simulink model "s_deng_rev1_13_sband"  (R2016b)
(part 4 of 69)

  flag_setup/5(in_reset_flags) -> pipeline36/1(d)
  pipeline36/1(q) -> edge_detect8/1(in)
  pipeline35/1(q) -> edge_detect9/1(in)
  pipeline34/1(q) -> [ndiode_flag]
  pipeline33/1(q) -> [adc_flag]
  pipeline32/1(q) -> [adc_count]
  start_flag_msw/1(in_reg) -> pipeline37/1(d)
  pipeline37/1(q) -> Concat4/1
  start_flag_lsw/1(in_reg) -> pipeline38/1(d)
  pipeline38/1(q) -> Concat4/2
  end_flag_msw/1(in_reg) -> pipeline39/1(d)
  pipeline39/1(q) -> Concat5/1
  end_flag_lsw/1(in_reg) -> pipeline40/1(d)
  pipeline40/1(q) -> Concat5/2
  pipeline54/1(q) -> [spead_data0]  "sp0_data"
  pipeline55/1(q) -> [spead_valid0]  "sp0_valid"
  pipeline56/1(q) -> [spead_eof0]  "sp0_eof"
  pipeline57/1(q) -> [spead_data1]  "sp1_data"
  pipeline58/1(q) -> [spead_valid1]  "sp1_valid"
  pipeline59/1(q) -> [spead_eof1]  "sp1_eof"
  pipeline60/1(q) -> [spead_data2]  "sp2_data"
  pipeline61/1(q) -> [spead_valid2]  "sp2_valid"
  pipeline62/1(q) -> [spead_eof2]  "sp2_eof"
  pipeline63/1(q) -> [spead_data3]  "sp3_data"
  pipeline64/1(q) -> [spead_valid3]  "sp3_valid"
  pipeline65/1(q) -> [spead_eof3]  "sp3_eof"
  pipeline97/1(q) -> Gateway Out70/1, pack_80_64_00/2(valid80)
  pipeline98/1(q) -> Gateway Out71/1, pack_80_64_00/3(word_start)
  pipeline99/1(q) -> Logical18/2, Gateway Out72/1, pack_80_64_00/4(pkt_start)
  pipeline101/1(q) -> Gateway Out73/1, pack_80_64_1/2(valid80)
  pipeline102/1(q) -> Gateway Out74/1, pack_80_64_1/3(word_start)
  pipeline105/1(q) -> Gateway Out76/1, pack_80_64_2/2(valid80)
  pipeline106/1(q) -> Gateway Out77/1, pack_80_64_2/3(word_start)
  pipeline109/1(q) -> Gateway Out79/1, pack_80_64_3/2(valid80)
  pipeline110/1(q) -> Gateway Out80/1, pack_80_64_3/3(word_start)
  pipeline112/1(q) -> Logical42/2, [rdy0], Gateway Out26/1
  pipeline113/1(q) -> Logical43/1, Gateway Out69/1, [vld0], Gateway Out25/1
  pipeline115/1(q) -> Logical11/2, [rdy1]
  pipeline116/1(q) -> Logical41/2, [vld1]
  pipeline118/1(q) -> Logical44/2, [rdy2]
  pipeline119/1(q) -> Logical45/1, [vld2]
  pipeline121/1(q) -> Logical46/2, [rdy3]
  pipeline122/1(q) -> Logical47/1, [vld3]
  Delay13/1 -> Logical8/1, Logical6/1
  Delay14/1 -> Logical7/2
  Delay15/1 -> Delay18/1
  Delay16/1 -> Delay19/1
  Delay17/1 -> Logical5/1
  Delay18/1 -> Delay20/1
  Delay19/1 -> Delay21/1
  Delay20/1 -> sample_masking/3(first_samples)
  Delay21/1 -> sample_masking/4(last_samples)
  Delay22/1 -> Logical3/2
  Delay23/1 -> Logical1/1
  Delay24/1 -> Delay25/1
  Delay25/1 -> Delay26/1
  Delay26/1 -> Delay27/1
  Delay27/1 -> sample_masking/1(timei)
  sample_masking/4(flag_valid) -> Delay28/1
  Delay28/1 -> [flag_en]
  Logical1/1 -> sample_masking/7(flag_en)  "flag_en"
  sample_masking/1(timeo) -> Delay29/1
  Delay29/1 -> [masked_time]
  [local_time] -> Delay30/1
  [en_armed] -> Delay31/1
  [local_time] -> Delay32/1, Delay34/1, Delay38/1, Delay40/1
  [start_time] -> Delay33/1
  [end_time] -> Delay35/1, Delay36/1
  Delay30/1 -> Delay24/1
  Delay31/1 -> Delay13/1
  Delay32/1 -> Relational3/1
  Delay33/1 -> Relational3/2
  Delay34/1 -> Relational4/1
  Delay35/1 -> Relational4/2
  Delay36/1 -> Relational5/1
  Delay37/1 -> Relational5/2
  Delay38/1 -> Relational6/1
  Delay39/1 -> Relational6/2
  Delay40/1 -> Relational7/1
  Delay41/1 -> Relational7/2
  Delay44/1 -> Logical4/1, Logical2/1
  Delay45/1 -> Relational/1
  Delay46/1 -> Relational/2
  Delay47/1 -> Relational1/1
  Delay48/1 -> Relational1/2
  Delay51/1 -> Relational2/1
  pipeline127/1(q) -> [pol0_always_on]
  [pol0_always_on] -> gbe0_traffic_control/1(always_on)
  [pol0_requested_pkts] -> gbe0_traffic_control/2(requested_pkts)
  [pol0_offset_data] -> gbe0_traffic_control/3(offset_data)
  [mrst] -> gbe0_traffic_control/4(mrst)
  [pol0_traffic_trigger] -> gbe0_traffic_control/5(traffic_trigger)
  gbe0_traffic_control/1(gbe_txen_gate) -> [gbe_txen_gate0]
  Constant68/1 -> pol1_sample_offset/1(sim_1)
  pipeline129/1(q) -> [pol1_offset_data]
  Constant67/1 -> pol0_sample_offset/1(sim_1)
  pipeline128/1(q) -> [pol0_offset_data]
  Constant69/1 -> pol0_num_pkts/1(sim_1)
  pipeline126/1(q) -> [pol0_requested_pkts]
  Constant73/1 -> pol1_num_pkts/1(sim_1)
  pipeline134/1(q) -> [pol1_requested_pkts]
  pipeline136/1(q) -> [pol1_always_on]
  pipeline5/1(q) -> [gbe_txen]
  Delay/1 -> pol_traffic_trigger/1(sim_1)
  Constant66/1 -> pol_tx_always_on/1(sim_1)
  Constant77/1 -> pol_tx_always_on/2(sim_2)
  pol0_num_pkts/1(in_pol0_num_pkts) -> pipeline126/1(d)
  pol1_num_pkts/1(in_pol1_num_pkts) -> pipeline134/1(d)
  pol_tx_always_on/1(in_pol0_tx_always_on) -> pipeline127/1(d)
  pol_tx_always_on/2(in_pol1_tx_always_on) -> pipeline136/1(d)
  pol0_sample_offset/1(in_pol0_sample_offset) -> pipeline128/1(d)
  pol1_sample_offset/1(in_pol1_sample_offset) -> pipeline129/1(d)
  Delay52/1 -> pol_traffic_trigger/2(sim_2)
  pol_traffic_trigger/1(in_pol0_tx_trigger) -> pipeline131/1(d)
  pipeline130/1(q) -> [pol1_traffic_trigger]
  pol_traffic_trigger/2(in_pol1_tx_trigger) -> pipeline130/1(d)
  edge_detect3/1(out) -> [cnt_rst]  "mrst"
  AddSub/1 -> Slice/1
  AddSub1/1 -> Slice1/1
  [tvg_stime] -> AddSub1/1, AddSub/1
  Constant81/1 -> speadtime0_offset/1(sim_1)
  Slice/1 -> Register5/1
  Slice1/1 -> Register6/1
  speadtime0_offset/1(in_speadtime_offset0) -> AddSub/2
  Constant82/1 -> speadtime1_offset/1(sim_1)
  speadtime1_offset/1(in_speadtime_offset1) -> AddSub1/2
  pipeline131/1(q) -> [pol0_traffic_trigger]
  gbe1_traffic_control/1(gbe_txen_gate) -> [gbe_txen_gate1]
  gbe2_traffic_control/1(gbe_txen_gate) -> [gbe_txen_gate2]
  gbe3_traffic_control/1(gbe_txen_gate) -> [gbe_txen_gate3]
  [spead_valid0] -> gbe0_traffic_control/6(spead_valid)
  [pol0_always_on] -> gbe1_traffic_control/1(always_on)
  [pol0_requested_pkts] -> gbe1_traffic_control/2(requested_pkts)
  [pol0_offset_data] -> gbe1_traffic_control/3(offset_data)
  [mrst] -> gbe1_traffic_control/4(mrst)
  [pol0_traffic_trigger] -> gbe1_traffic_control/5(traffic_trigger)
  [pol1_always_on] -> gbe2_traffic_control/1(always_on)
  [pol1_requested_pkts] -> gbe2_traffic_control/2(requested_pkts)
  [pol1_offset_data] -> gbe2_traffic_control/3(offset_data)
  [mrst] -> gbe2_traffic_control/4(mrst)
  [pol1_traffic_trigger] -> gbe2_traffic_control/5(traffic_trigger)
  [pol1_always_on] -> gbe3_traffic_control/1(always_on)
  [pol1_requested_pkts] -> gbe3_traffic_control/2(requested_pkts)
  [pol1_offset_data] -> gbe3_traffic_control/3(offset_data)
  [mrst] -> gbe3_traffic_control/4(mrst)
  [pol1_traffic_trigger] -> gbe3_traffic_control/5(traffic_trigger)
  [spead_valid1] -> gbe1_traffic_control/6(spead_valid)
  [spead_valid2] -> gbe2_traffic_control/6(spead_valid)
  [spead_valid3] -> gbe3_traffic_control/6(spead_valid)
  Constant59/1 -> Delay/1
  Constant40/1 -> Delay52/1
  master_reset_sim7/1 -> dram_addr_offset/1(sim_1)
  master_reset_sim8/1 -> arb_rst/1(sim_1)
  master_reset_sim9/1 -> arb_en/1(sim_1)
  pipeline133/1(q) -> [arb_en0]
  pipeline138/1(q) -> [dram_addr_offset0]
  master_reset_sim1/1 -> dram_read_length/1(sim_1)
  master_reset_sim2/1 -> dram_rd_trigger/1(sim_1)
  pipeline150/1(q) -> [dram_rd_trig0]
  master_reset_sim3/1 -> dram_tvg/1(sim_1)
  master_reset_sim4/1 -> dram_tvg_length/1(sim_1)
  pipeline148/1(q) -> [dram_tvg_length0]
  edge_detect13/1(out) -> [arb_rst0]
  pipeline135/1(q) -> edge_detect13/1(in)
  master_reset_sim5/1 -> dram_rd_repeat/1(sim_1)
  pipeline151/1(q) -> [dram_rd_repeat0]
  pipeline146/1(q) -> Slice13/1, Slice11/1
  Slice13/1 -> Logical17/1, [tvg_sel0]
  Slice11/1 -> Logical17/2
  Logical17/1 -> [dram_tvg0]
  pipeline149/1(q) -> [dram_read_length0]
  master_reset_sim6/1 -> dram_rd_repeat_rate/1(sim_1)
  pipeline137/1(q) -> [dram_rd_repeat_delay0]
  [cwg_80_0] -> pipeline190/1(d)
  pipeline158/1(q) -> [source_sel_0]
  pipeline159/1(q) -> [source_sel_1]
  Constant87/1 -> src_sel_cntrl/1(sim_1)
  Constant88/1 -> src_sel_cntrl/2(sim_2)
  src_sel_cntrl/1(in_src_sel_0) -> pipeline158/1(d)
  src_sel_cntrl/2(in_src_sel_1) -> pipeline159/1(d)
  [source_sel_0] -> pipeline189/1(d)
  Inverter/1 -> fifo1/2(fifo_we_en)
  Gateway Out24/1 -> To Workspace24/1
  Slice23/1 -> Gateway Out24/1
  Gateway Out25/1 -> To Workspace25/1
  Gateway Out26/1 -> To Workspace26/1
  dram_rd_repeat_rate/1(in_dram_rd_repeat_rate) -> pipeline137/1(d)
  dram_rd_repeat/1(in_dram_rd_repeat) -> pipeline151/1(d)
  dram_tvg/1(in_arb_tvg) -> pipeline146/1(d)
  dram_tvg_length/1(in_tvg_length) -> pipeline148/1(d)
  dram_addr_offset/1(in_dram_addr_offset) -> pipeline138/1(d)
  dram_read_length/1(in_dram_read_length) -> pipeline149/1(d)
  dram_rd_trigger/1(in_arb_trig) -> pipeline150/1(d)
  arb_en/1(in_arb_en) -> pipeline133/1(d)
  arb_rst/1(in_rst) -> pipeline135/1(d)
  pipeline189/1(q) -> Mux5/1
  pipeline190/1(q) -> Mux5/2
  pipeline191/1(q) -> Mux5/3
  [adc_count] -> Concat6/1
  Constant90/1 -> Concat6/2
  Delay4/1 -> [status0]
  Delay55/1 -> [status3]
  Delay54/1 -> [status2]
  Delay53/1 -> [status1]
  Concat6/1 -> Delay55/1, Delay4/1, Delay53/1, Delay54/1
  [ndiode_flag] -> Convert28/1
  Logical/1 -> Convert27/1
  Logical19/1 -> Convert30/1
  [adc_flag] -> Convert29/1
  [flag_en] -> Logical/1, Logical19/2
  Convert28/1 -> Logical/2
  Convert29/1 -> Logical19/1
  Convert30/1 -> Concat6/3
  Convert27/1 -> Concat6/4
  Gateway Out13/1 -> To Workspace13/1
  [local_time] -> pipeline203/1(d)
  [mrst] -> pipeline201/1(d)
  [wng_man_rst0] -> pipeline199/1(d)
  wng_rst/1(wng_rst) -> Gateway Out13/1, [wng_rst0]
  Constant89/1 -> rpt_length_wng0/1(sim_1)
  pipeline200/1(q) -> wng_rst/5(num_samples_for_rst)
  pipeline199/1(q) -> wng_rst/4(man_rst)
  pipeline201/1(q) -> wng_rst/3(mrst)
  pipeline202/1(q) -> wng_rst/2(future_time)
  pipeline203/1(q) -> wng_rst/1(local_time)
  Constant95/1 -> rpt_load_time_msw_wng0/1(sim_1)
  Constant93/1 -> rpt_load_time_lsw_wng0/1(sim_1)
  Concat3/1 -> Delay1/1
  pipeline204/1(q) -> Concat3/1
  pipeline205/1(q) -> Concat3/2
  rpt_load_time_lsw_wng0/1(in_reg) -> pipeline205/1(d)
  rpt_load_time_msw_wng0/1(in_reg) -> pipeline204/1(d)
  Delay1/1 -> pipeline202/1(d)
  rpt_length_wng0/1(in_samples) -> pipeline206/1(d)
  pipeline206/1(q) -> pipeline200/1(d)
  [local_time] -> pipeline154/1(d)
  impulse/1(impulse0) -> [impulse_gen0]
  pipeline152/1(q) -> impulse/2(future_time)
  pipeline154/1(q) -> impulse/1(local_time)
  Constant92/1 -> impulse_load_time_msw/1(sim_1)
  Constant91/1 -> impulse_load_time_lsw/1(sim_1)
  Concat7/1 -> Delay10/1
  pipeline155/1(q) -> Concat7/1
  pipeline160/1(q) -> Concat7/2
  impulse_load_time_lsw/1(in_reg) -> pipeline160/1(d)
  impulse_load_time_msw/1(in_reg) -> pipeline155/1(d)
  Delay10/1 -> pipeline152/1(d)
  pipeline163/1(q) -> Mux5/4
  [impulse_gen0] -> pipeline163/1(d)
  gpio/1 -> Terminator62/1
  Gateway Out/1 -> To Workspace/1
  impulse/2(impulse_gpio) -> [impulse_gpio]
  pipeline145/1(q) -> impulse/3(delay_correction)
  impulse_delay_correction/1(in_reg) -> pipeline145/1(d)
  Constant55/1 -> impulse_delay_correction/1(sim_1)
  pipeline144/1(q) -> Gateway Out/1, gpio/1
  [impulse_gpio] -> pipeline144/1(d)
  bus_create4/1(bus_out) -> pipeline191/1(d)
  [tvg_ltime] -> Delay11/1
  Delay11/1 -> Delay12/1
  [data_80_0] -> Delay56/1
  Delay56/1 -> Delay57/1
  bus_expand14/7(out2) -> pipeline167/1(d)
  bus_expand14/8(lsb_out1) -> pipeline170/1(d)
  bus_expand14/6(out3) -> pipeline171/1(d)
  bus_expand14/5(out4) -> pipeline172/1(d)
  bus_expand14/4(out5) -> pipeline209/1(d)
  bus_expand14/3(out6) -> pipeline210/1(d)
  bus_expand14/2(out7) -> pipeline211/1(d)
  bus_expand14/1(msb_out8) -> pipeline212/1(d)
  pipeline212/1(q) -> ss_fifo_in/1(in_d0)
  pipeline211/1(q) -> ss_fifo_in/2(in_d1)
  pipeline210/1(q) -> ss_fifo_in/3(in_d2)
  pipeline209/1(q) -> ss_fifo_in/4(in_d3)
  pipeline172/1(q) -> ss_fifo_in/5(in_d4)
  pipeline171/1(q) -> ss_fifo_in/6(in_d5)
  pipeline167/1(q) -> ss_fifo_in/7(in_d6)
  pipeline170/1(q) -> ss_fifo_in/8(in_d7)
  Delay57/1 -> bus_expand14/1(bus_in)
  Delay12/1 -> pipeline215/1(d), Relational8/1
  pipeline215/1(q) -> ss_localtime/1(in_time)
  pipeline213/1(q) -> ss_fifo_in/9(in_gpio_trig)
  Delay58/1 -> Delay59/1
  Delay59/1 -> pipeline213/1(d)
  [impulse_gpio] -> Delay60/1
  Delay60/1 -> Delay58/1
  pipeline214/1(q) -> impulse/4(Impulse_offset)
  Constant109/1 -> impulse_offset/1(sim_1)
  impulse_offset/1(in_reg) -> pipeline214/1(d)
  Constant108/1 -> ss_trig_time_msw/1(sim_1)
  Constant107/1 -> ss_trig_time_lsw/1(sim_1)
  Concat8/1 -> Delay61/1
  pipeline216/1(q) -> Concat8/1
  pipeline217/1(q) -> Concat8/2
  ss_trig_time_lsw/1(in_reg) -> pipeline217/1(d)
  ss_trig_time_msw/1(in_reg) -> pipeline216/1(d)
  Delay61/1 -> Relational8/2
  Relational8/1 -> edge_detect/1
  pipeline218/1(q) -> ss_fifo_in/10(we)
  [fifoselect] -> pipeline219/1(d), pipeline218/1(d)
  pipeline219/1(q) -> ss_localtime/2(we)
  edge_detect/1 -> ss_localtime/3(trig), ss_fifo_in/11(trig)
  Constant111/1 -> start_load_time_msw/1(sim_1)
  Constant110/1 -> start_load_time_lsw/1(sim_1)
  pipeline220/1(q) -> Concat9/1
  pipeline221/1(q) -> Concat9/2
  start_load_time_msw/1(in_reg) -> pipeline220/1(d)
  start_load_time_lsw/1(in_reg) -> pipeline221/1(d)
  Concat9/1 -> Delay62/1
  Constant113/1 -> stop_load_time_msw/1(sim_1)
  Constant112/1 -> stop_load_time_lsw/1(sim_1)
  pipeline222/1(q) -> Concat10/1
  pipeline223/1(q) -> Concat10/2
  stop_load_time_msw/1(in_reg) -> pipeline222/1(d)
  stop_load_time_lsw/1(in_reg) -> pipeline223/1(d)
  Concat10/1 -> Delay63/1
  Delay62/1 -> pipeline225/1(d)
  Delay63/1 -> pipeline224/1(d)
  pipeline225/1(q) -> start_stop_cntrl/1(start_time)
  pipeline224/1(q) -> start_stop_cntrl/2(stop_time)
  [mrst] -> start_stop_cntrl/3(rst)
  start_stop_cntrl/1(start_stop_sel) -> [start_stop_sel]
  pipeline195/1(q) -> Mux3/2
  Mux3/1 -> [data_80_0]
  [start_stop_sel] -> Mux3/1
  Constant115/1 -> Mux3/3
  data_ins/1(data) -> Delay73/1
  debug_control/1(in_reg) -> Slice2/1, Slice10/1
  Constant94/1 -> debug_control/1(sim_1)
  Constant120/1 -> pkt_size0/1(sim_1)
  pkt_size0/1(in_reg) -> Delay67/1, Relational9/1
  pkt_size_calc0/1(en_out) -> Delay69/1
  pkt_size_calc0/2(eof) -> Delay70/1
  data_ins/2(en_out) -> Delay74/1
  data_ins/3(eof_out) -> Delay75/1
  [debug_cnt_rst] -> data_ins/1(rst)
  Slice2/1 -> Delay64/1
  Delay64/1 -> [debug_cnt_rst]
  Gateway Out8/1 -> Scope1/1
  Gateway Out10/1 -> Scope1/2
  Gateway Out11/1 -> Scope1/3
  Gateway Out14/1 -> Scope1/4
  Slice3/1 -> Gateway Out8/1
  Slice4/1 -> Gateway Out10/1
  Logical22/1 -> Counter1/2, Gateway Out7/1
  Counter1/1 -> Delay68/1, Gateway Out2/1
  [debug_cnt_rst] -> Counter1/1
  Delay67/1 -> pkt_size_calc0/2(size)
  Delay68/1 -> Convert10/1
  Delay69/1 -> data_ins/2(en_in)
  Delay70/1 -> data_ins/3(eof_in)
  Delay71/1 -> pkt_size_calc0/3(en_in)
  Delay73/1 -> Slice3/1, Slice4/1
  Delay74/1 -> Gateway Out11/1, Logical22/1
  Delay75/1 -> Gateway Out14/1, Logical22/2
  Slice10/1 -> Delay81/1
  pkt_rate0/1(en) -> Delay83/1, Logical23/3
  Logical23/1 -> Delay71/1
  Delay81/1 -> Logical23/2
  Gateway Out2/1 -> Scope4/1
  Gateway Out7/1 -> Scope4/2
  Counter3/1 -> Delay82/1
  Delay82/1 -> debug_rate/1(out_reg)
  Delay83/1 -> Counter3/1
  Constant119/1 -> Relational9/2
  Relational9/1 -> Logical23/1
  [debug_cnt_rst] -> pkt_size_calc0/1(rst)
  Convert10/1 -> debug_tx_pkt_cnt/1(out_reg)
  [forty_gbe_led_up] -> Delay72/1
  [forty_gbe_led_rx] -> Delay101/1
  [forty_gbe_led_tx] -> Delay110/1
  [forty_gbe_tx_afull] -> Delay107/1
  [forty_gbe_tx_overflow] -> Delay112/1
  [forty_gbe_rx_overrun] -> Delay111/1
  [arb_rst0] -> Terminator9/1
  [arb_en0] -> Terminator10/1
  [dram_rd_repeat0] -> Terminator11/1
  [dram_rd_repeat_delay0] -> Terminator13/1
  [tvg_sel0] -> Terminator14/1
  [dram_tvg0] -> Terminator17/1
  [dram_tvg_length0] -> Terminator19/1
  [dram_addr_offset0] -> Terminator21/1
  [dram_read_length0] -> Terminator22/1
  Delay107/1 -> status0/4(out_tx_afull)
  Delay101/1 -> status0/2(out_led_rx)
  Delay112/1 -> status0/5(out_tx_overflow)
  Delay111/1 -> status0/6(out_rx_overrun)
  Delay110/1 -> status0/3(out_led_tx)
  Delay72/1 -> status0/1(out_led_up)
  pipeline15/1(q) -> [gbe_port]
  Constant26/1 -> [spead_heapsize]
  Constant27/1 -> [spead_pktlen]
  Constant45/1 -> [spead_heapoffset]
  Constant8/1 -> [adc_data_offset]
  [spead_data0] -> pipeline72/1(d)
  [spead_valid0] -> pipeline73/1(d)
  wr_addr0/1 -> Gateway Out63/1, 64_to_256/1  "waddr"
  [spead_valid0] -> Gateway Out19/1, edge_detect27/1(in), edge_detect7/1, pipeline67/1(d)
  Constant116/1 -> 64_to_256/6
  Constant121/1 -> 64_to_256/5
  rd_addr0/1 -> Gateway Out64/1, 64_to_256/4, Relational13/2  "rdaddr"
  edge_detect7/1 -> wr_addr0/1
  pipeline67/1(q) -> wr_addr0/2
  pipeline72/1(q) -> 64_to_256/2
  pipeline73/1(q) -> 64_to_256/3  "dv64_0"
  64_to_256/1 -> Terminator25/1
  edge_detect27/1(out) -> rd_addr0/1, rd_arm/3, rd_arm/1
  Constant131/1 -> Relational13/1
  Relational13/1 -> rd_arm/2  "rd_done"
  rd_arm/1 -> pipeline74/1(d), rd_addr0/2  "rd_en"
  edge_detect17/1(out) -> [sp256_eof0]  "eof256_0"
  [spead_data2] -> pipeline77/1(d)
  [spead_valid2] -> pipeline80/1(d)
  wr_addr2/1 -> 64_to_1/1  "waddr"
  [spead_valid2] -> pipeline76/1(d), edge_detect18/1, edge_detect20/1(in), Gateway Out21/1
  Constant21/1 -> 64_to_1/6
  Constant25/1 -> 64_to_1/5
  rd_addr2/1 -> Relational14/2, 64_to_1/4  "rdaddr"
  edge_detect18/1 -> wr_addr2/1
  pipeline76/1(q) -> wr_addr2/2
  pipeline77/1(q) -> 64_to_1/2
  pipeline80/1(q) -> 64_to_1/3  "dv64_2"
  64_to_1/1 -> Terminator26/1
  edge_detect20/1(out) -> rd_addr2/1
  Constant86/1 -> Relational14/1
  Relational14/1 -> rd_arm2/2  "rd_done"
  rd_arm2/1 -> rd_addr2/2, pipeline81/1(d)  "rd_en"
  pipeline81/1(q) -> edge_detect19/1(in), pipeline82/1(d)  "dv256"
  edge_detect19/1(out) -> [sp256_eof2]  "eof256_2"
  pipeline82/1(q) -> [sp256_dv2]  "dv256_2"
  [sp256_eof0] -> rd_arm2/3, rd_arm2/1
  [spead_data1] -> pipeline84/1(d)
  [spead_valid1] -> pipeline85/1(d)
  wr_addr1/1 -> 64_to_2/1  "waddr"
  [spead_valid1] -> pipeline83/1(d), edge_detect21/1, Gateway Out20/1, edge_detect23/1(in)
  Constant122/1 -> 64_to_2/6
  Constant123/1 -> 64_to_2/5
  rd_addr1/1 -> Relational10/2, 64_to_2/4  "rdaddr"
  edge_detect21/1 -> wr_addr1/1
  pipeline83/1(q) -> wr_addr1/2
  pipeline84/1(q) -> 64_to_2/2
  pipeline85/1(q) -> 64_to_2/3  "dv64_1"
  64_to_2/1 -> Terminator27/1
  edge_detect23/1(out) -> rd_arm1/3, rd_arm1/1, rd_addr1/1
  Constant124/1 -> Relational10/1
  Relational10/1 -> rd_arm1/2  "rd_done"
  rd_arm1/1 -> rd_addr1/2, pipeline86/1(d)  "rd_en"
  pipeline86/1(q) -> edge_detect22/1(in), pipeline124/1(d)  "dv256"
  edge_detect22/1(out) -> [sp256_eof1]  "eof256_1"
  pipeline124/1(q) -> [sp256_dv1]  "dv256_1"
  [spead_data3] -> pipeline132/1(d)
  [spead_valid3] -> pipeline139/1(d)
  wr_addr3/1 -> 64_to_3/1  "waddr"
  [spead_valid3] -> edge_detect26/1(in), Gateway Out22/1, edge_detect24/1, pipeline125/1(d)
  Constant125/1 -> 64_to_3/6
  Constant126/1 -> 64_to_3/5
  rd_addr3/1 -> 64_to_3/4, Relational11/2  "rdaddr"
  edge_detect24/1 -> wr_addr3/1
  pipeline125/1(q) -> wr_addr3/2
  pipeline132/1(q) -> 64_to_3/2
  pipeline139/1(q) -> 64_to_3/3  "dv64_3"
  64_to_3/1 -> Terminator24/1
  edge_detect26/1(out) -> rd_addr3/1
  Constant127/1 -> Relational11/1
  Relational11/1 -> rd_arm3/2  "rd_done"
  rd_arm3/1 -> pipeline140/1(d), rd_addr3/2  "rd_en"
  pipeline140/1(q) -> edge_detect25/1(in), pipeline141/1(d)  "dv256"
  edge_detect25/1(out) -> [sp256_eof3]  "eof256_3"
  pipeline141/1(q) -> [sp256_dv3]  "dv256_3"
  [sp256_eof1] -> rd_arm3/1, rd_arm3/3
  [gbe_txen0] -> Logical12/2
  pipeline75/1(q) -> [sp256_dv0]  "dv256_0"
  [sp256_eof0] -> Logical12/1
  [sp256_dv0] -> Logical13/1
  [gbe_txen0] -> Logical13/2
  Logical13/1 -> Gateway Out65/1, [sp256_dvg0]
  Logical12/1 -> Gateway Out90/1, [sp256_eofg0]
  [gbe_txen1] -> Logical14/2
  [sp256_eof1] -> Logical14/1
  [sp256_dv1] -> Logical15/1
  [gbe_txen1] -> Logical15/2
  Logical15/1 -> Gateway Out66/1, [sp256_dvg1]
  Logical14/1 -> Gateway Out89/1, [sp256_eofg1]
  [gbe_txen2] -> Logical16/2
  [sp256_eof2] -> Logical16/1
  [sp256_dv2] -> Logical25/1
  [gbe_txen2] -> Logical25/2
  Logical25/1 -> Gateway Out67/1, [sp256_dvg2]
  Logical16/1 -> Gateway Out88/1, [sp256_eofg2]
  [gbe_txen3] -> Logical26/2
  [sp256_eof3] -> Logical26/1
  [sp256_dv3] -> Logical27/1
  [gbe_txen3] -> Logical27/2
  Logical27/1 -> Gateway Out68/1, [sp256_dvg3]
  Logical26/1 -> Gateway Out87/1, [sp256_eofg3]
  [sel_munge] -> Mux17/1
  Mux17/1 -> [sp256_data3]
  [sel_munge] -> Mux16/1
  Mux16/1 -> [sp256_data2]
  [sel_munge] -> Mux18/1
  Mux18/1 -> [sp256_data1]
  [sel_munge] -> Mux19/1
  Mux19/1 -> [sp256_data0]
  [gbe_rst] -> pipeline233/1(d)
  Constant18/1 -> forty_gbe/7(rx_ack)
  Constant56/1 -> forty_gbe/8(rx_overrun_ack)
  pipeline239/1(q) -> forty_gbe/9(debug_rst)
  Logical40/1 -> pipeline238/1(d)
  Logical39/1 -> pipeline235/1(d)
  [sp256_data] -> pipeline234/1(d)
  [gbe_port] -> pipeline237/1(d)
  [gbe_txip] -> pipeline236/1(d)
  forty_gbe/1(led_up) -> pipeline178/1(d)
  forty_gbe/2(led_rx) -> pipeline87/1(d)
  forty_gbe/3(led_tx) -> pipeline176/1(d)
  forty_gbe/4(tx_afull) -> pipeline177/1(d)
  forty_gbe/5(tx_overflow) -> pipeline179/1(d)
  forty_gbe/12(rx_overrun) -> pipeline197/1(d)
  forty_gbe/6(rx_data) -> Terminator42/1
  forty_gbe/7(rx_valid) -> Terminator43/1
  forty_gbe/10(rx_end_of_frame) -> Terminator44/1
  forty_gbe/11(rx_bad_frame) -> Terminator45/1
  forty_gbe/8(rx_source_ip) -> Terminator7/1
  forty_gbe/9(rx_source_port) -> Terminator8/1
  pipeline178/1(q) -> [forty_gbe_led_up]
  pipeline87/1(q) -> [forty_gbe_led_rx]
  pipeline176/1(q) -> [forty_gbe_led_tx]
  pipeline177/1(q) -> [forty_gbe_tx_afull]
  pipeline179/1(q) -> [forty_gbe_tx_overflow]
  pipeline197/1(q) -> [forty_gbe_rx_overrun]
  forty_gbe/14(rx_dest_port) -> Terminator40/1
  forty_gbe/13(rx_dest_ip) -> Terminator41/1
  [gbe_txen] -> Logical39/1
  [sp256_dv] -> Logical39/2
  [gbe_txen] -> Logical40/1
  [sp256_eof] -> Logical40/2
  pipeline233/1(q) -> forty_gbe/1(rst)
  pipeline234/1(q) -> forty_gbe/2(tx_data)
  pipeline235/1(q) -> forty_gbe/3(tx_valid)
  pipeline236/1(q) -> forty_gbe/4(tx_dest_ip)
  pipeline237/1(q) -> forty_gbe/5(tx_dest_port)
  pipeline238/1(q) -> forty_gbe/6(tx_end_of_frame)
  [cnt_rst] -> pipeline239/1(d)
  ramp0/1 -> [rampdata0]
  [vld0] -> ramp0/2
  [rdy0] -> ramp0/1
  ramp1/1 -> [rampdata1]
  [vld1] -> ramp1/2
  [rdy1] -> ramp1/1
  [spead_data0] -> spead_snap0/1(in_d64)
  [spead_valid0] -> spead_snap0/2(we)
  [spead_eof0] -> spead_detail/1(in_eof)
  [spead_valid0] -> spead_detail/2(in_we), spead_detail/3(we)
  Logical9/1 -> spead_detail/4(trig), spead_snap0/3(trig)
  [spead_eof0] -> Logical9/2
  [speadsnap_arm] -> Logical9/1
  speadsnap_control/1(in_speadsnap_arm) -> Delay65/1
  Delay65/1 -> [speadsnap_arm]
  ramp2/1 -> [rampdata2]
  [vld2] -> ramp2/2
  [rdy2] -> ramp2/1
  ramp3/1 -> [rampdata3]
  [vld3] -> ramp3/2
  [rdy3] -> ramp3/1
  ramp80/1 -> [ramp79]
  [rst_ramp80] -> ramp80/1
  Delay76/1 -> [sel_ramp80]
  ramp_control/1(in_sel_ramp80) -> Delay76/1
  Delay77/1 -> [rst_ramp80]
  ramp_control/2(in_rst_ramp80) -> Delay77/1
  Delay66/1 -> [sel_munge]
  ramp_control/3(in_sel_munge) -> Delay66/1
  gbe_control/1(in_gbe0) -> [gbe_txen0]
  gbe_control/2(in_gbe1) -> [gbe_txen1]
  gbe_control/3(in_gbe2) -> [gbe_txen2]
  gbe_control/4(in_gbe3) -> [gbe_txen3]
  Constant117/1 -> gbe_control/2(sim_2)
  Constant65/1 -> gbe_control/1(sim_1)
  Constant118/1 -> gbe_control/3(sim_3)
  Constant132/1 -> gbe_control/4(sim_4)
  pipeline68/1(q) -> Mux14/2
  [sel_ramp80] -> Mux14/1
  Mux14/1 -> Slice23/1, Gateway Out107/1, spead_pack0/3(data64)
  pack_80_64_00/3(data64) -> pipeline68/1(d)  "d64_00"
  [sel_ramp80] -> Mux15/1
  Mux15/1 -> Gateway Out108/1, spead_pack1/3(data64)
  [sel_ramp80] -> Mux20/1
  Mux20/1 -> Gateway Out109/1, spead_pack2/3(data64)
  [sel_ramp80] -> Gateway Out113/1, Mux21/1
  [ramp79] -> bus_create4/2(in2)  "d80_0"
  Constant133/1 -> bus_create4/1(in1)
  [rampdata0] -> Mux14/3
  [rampdata1] -> Mux15/3
  pipeline117/1(q) -> Mux15/2
  [rampdata2] -> Mux20/3
  pipeline120/1(q) -> Mux20/2
  [rampdata3] -> Mux21/3
  pipeline123/1(q) -> Mux21/2
  Logical11/1 -> spead_pack1/1(data64_ready)
  Logical41/1 -> spead_pack1/2(data64_valid), Gateway Out62/1
  [gbe_txen_gate1] -> Logical41/1, Logical11/1
  [gbe_txen_gate0] -> Logical43/2, Gateway Out60/1, Logical42/1
  Logical43/1 -> Gateway Out61/1, spead_pack0/2(data64_valid)
  Logical42/1 -> spead_pack0/1(data64_ready)
  [gbe_txen_gate2] -> Logical45/2, Logical44/1
  Logical44/1 -> spead_pack2/1(data64_ready)
  Logical45/1 -> spead_pack2/2(data64_valid), Gateway Out85/1
  [gbe_txen_gate3] -> Logical47/2, Logical46/1
  Logical46/1 -> spead_pack3/1(data64_ready)
  Logical47/1 -> spead_pack3/2(data64_valid), Gateway Out86/1
  bram_munge0/1(Out1) -> Mux19/2
  bram_munge1/1(Out1) -> Mux18/2
  bram_munge2/1(Out1) -> Mux16/2
  bram_munge3/1(Out1) -> Mux17/2
  Delay78/1 -> Mux9/1
  [speadtime0] -> Mux9/3
  pipeline96/1(q) -> Mux9/2
  Mux9/1 -> pack_80_64_00/1(data80)
  Logical18/1 -> Delay78/1
  [sel_insert_time] -> Logical18/1
  [mrst] -> Gateway Out98/1, ticks_since_mrst/1(reset)
  [msync] -> Gateway Out99/1, ticks_since_mrst/2(sync)
  control/1(in_cnt_rst) -> pipeline/1(d)
  ramp_control/4(in_sel_insert_time) -> Delay79/1
  Delay79/1 -> [sel_insert_time]
  pipeline103/1(q) -> Logical48/2, Gateway Out75/1, pack_80_64_1/4(pkt_start)
  Delay80/1 -> Mux10/1
  Logical48/1 -> Delay80/1
  [sel_insert_time] -> Logical48/1
  [speadtime1] -> Mux10/3
  pipeline100/1(q) -> Mux10/2
  Mux10/1 -> pack_80_64_1/1(data80)
  Delay84/1 -> Mux22/1
  Logical49/1 -> Delay84/1
  [sel_insert_time] -> Logical49/1
  Mux22/1 -> pack_80_64_2/1(data80)
  [speadtime0] -> Mux22/3
  pipeline104/1(q) -> Mux22/2
  pipeline111/1(q) -> Logical50/2, Gateway Out81/1, pack_80_64_3/4(pkt_start)
  Delay85/1 -> Mux23/1
  Logical50/1 -> Delay85/1
  [sel_insert_time] -> Logical50/1
  Mux23/1 -> pack_80_64_3/1(data80)
  [speadtime1] -> Mux23/3
  pipeline108/1(q) -> Mux23/2
  [start_stop_sel] -> Counter4/2
  Counter4/1 -> start_stop_ctr/1(out_reg)
  [cnt_rst] -> Counter4/1
  [gbe_txen_gate0] -> Counter5/2
  Counter5/1 -> tx_gate_ctrs/1(out_sp0)
  [cnt_rst] -> Counter6/1, Counter7/1, Counter8/1, Counter5/1
  Counter6/1 -> tx_gate_ctrs/2(out_sp1)
  Counter7/1 -> tx_gate_ctrs/3(out_sp2)
  Counter8/1 -> tx_gate_ctrs/4(out_sp3)
  [gbe_txen_gate3] -> Counter8/2
  [gbe_txen_gate2] -> Counter7/2
  [gbe_txen_gate1] -> Counter6/2
  Mux5/1 -> pipeline195/1(d)
  [cwg_80_1] -> pipeline114/1(d)
  [source_sel_1] -> pipeline71/1(d)
  pipeline71/1(q) -> Mux25/1
  pipeline114/1(q) -> Mux25/2
  pipeline142/1(q) -> Mux25/3
  pipeline70/1(q) -> Mux25/4
  [impulse_gen0] -> pipeline70/1(d)
  bus_create5/1(bus_out) -> pipeline142/1(d)
  pipeline143/1(q) -> Mux6/2
  [start_stop_sel] -> Mux6/1
  Constant20/1 -> Mux6/3
  [ramp79] -> bus_create5/2(in2)  "d80_0"
  Constant24/1 -> bus_create5/1(in1)
  Mux25/1 -> pipeline143/1(d)
  scale_wng1/1(in_scale) -> Gateway Out6/1, pipeline47/1(d)
  scale_wng_corr/1(in_scale) -> pipeline46/1(d)
  [wng0_tp0] -> pipeline91/1(d)
  [wng1_tp0] -> pipeline94/1(d)
  cwg_corr/1(bus_out) -> pipeline90/1(d)
  bus_addsub2/1(dout) -> Delay8/1
  bus_addsub4/1(dout) -> bus_convert6/1(din)
  bus_mult/1(a*b) -> [cwg0_tp1], bus_convert/1(din)
  bus_addsub5/1(dout) -> bus_convert7/1(din)
  bus_mult1/1(a*b) -> bus_convert1/1(din), [cwg1_tp1]
  scale_out1/1(in_scale) -> Gateway Out3/1, pipeline79/1(d)
  Constant1/1 -> scale_wng_corr/1(sim_1)
  pipeline45/1(q) -> [wng_scale0]
  pipeline46/1(q) -> [wng_scale_corr]
  pipeline47/1(q) -> [wng_scale1]
  Delay8/1 -> bus_convert4/1(din)
  Delay139/1 -> bus_addsub4/1(a)
  Delay9/1 -> bus_addsub5/1(a)
  Delay86/1 -> bus_addsub5/2(b)
  pipeline88/1(q) -> bus_mult1/1(a), [cwg1_tp0]
  pipeline79/1(q) -> bus_mult1/2(b)
  pipeline78/1(q) -> bus_mult/2(b)
  pipeline91/1(q) -> bus_addsub/1(a)
  pipeline92/1(q) -> bus_addsub/2(b)
  pipeline93/1(q) -> bus_addsub1/1(a)
  [wng_corr_tp0] -> pipeline93/1(d), pipeline92/1(d)
  pipeline94/1(q) -> bus_addsub1/2(b)
  [cwg_corr] -> bus_addsub2/2(b)
  pipeline156/1(q) -> [cwg_80_0]
  pipeline157/1(q) -> [cwg_80_1]
  Delay5/1 -> bus_addsub4/2(b)
  bus_convert/1(dout) -> [cwg0_tp2], pipeline156/1(d)
  bus_convert2/1(dout) -> [wng_sum0]
  bus_convert3/1(dout) -> [wng_sum1]
  bus_convert4/1(dout) -> [cwg_corr_out0]
  bus_convert5/1(dout) -> [cwg_corr_out1]
  bus_convert6/1(dout) -> pipeline53/1(d)
  bus_convert7/1(dout) -> pipeline88/1(d)
  Constant32/1 -> scale_wng1/1(sim_1)
  scale_wng0/1(in_scale) -> Gateway Out17/1, pipeline45/1(d)
  scale_out0/1(in_scale) -> Gateway Out5/1, pipeline78/1(d)
  Constant64/1 -> freq_cwg0/1(sim_1)
  scale_cwg0/1(in_scale) -> pipeline48/1(d)
  freq_cwg0/1(in_frequency) -> pipeline49/1(d)
  Constant79/1 -> freq_cwg_corr/1(sim_1)
  freq_cwg_corr/1(in_frequency) -> pipeline51/1(d)
  scale_cwg_corr/1(in_scale) -> pipeline50/1(d)
  Constant80/1 -> scale_cwg_corr/1(sim_1)
  Constant58/1 -> scale_out1/1(sim_1)
  Constant57/1 -> scale_out0/1(sim_1)
  pipeline49/1(q) -> cwg0/1(freq)
  pipeline48/1(q) -> cwg0/2(scale)
  [mrst] -> pipeline180/1(d)
  Constant62/1 -> rpt_length_cwg0/1(sim_1)
  rpt_en_cwg0/1(in_en) -> Convert25/1
  Constant70/1 -> rpt_en_cwg0/1(sim_1)
  Convert25/1 -> pipeline181/1(d)
  cwg0/1(bus_out) -> pipeline95/1(d)
  rpt_length_cwg0/1(in_repeat_length) -> pipeline182/1(d)
  pipeline180/1(q) -> cwg0/3(rst)
  pipeline181/1(q) -> cwg0/4(repeat_en)
  pipeline182/1(q) -> cwg0/5(repeat_length)
  cwg0/3(rpt_rst) -> Terminator61/1
  Constant28/1 -> man_rst_wng0/1(sim_1)
  Logical20/1 -> pipeline198/1(d)
  man_rst_wng0/1(in_rst) -> [wng_man_rst0], Logical20/2
  [wng_rst0] -> Logical20/1
  pipeline51/1(q) -> cwg_corr/1(freq)
  pipeline50/1(q) -> cwg_corr/2(scale)
  pipeline147/1(q) -> cwg_corr/3(rst)
  pipeline161/1(q) -> cwg_corr/4(repeat_en)
  pipeline162/1(q) -> cwg_corr/5(repeat_length)
  Constant96/1 -> cwg_corr/6(en)
  [mrst] -> pipeline147/1(d)
  rpt_en_cwg_corr/1(in_en) -> pipeline161/1(d)
  cwg_corr/3(rpt_rst) -> Terminator64/1
  cwg_corr/2(dvalid) -> Terminator65/1
  Constant97/1 -> rpt_en_cwg_corr/1(sim_1)
  rpt_length_cwg_corr/1(in_repeat_length) -> pipeline162/1(d)
  Constant99/1 -> rpt_length_cwg_corr/1(sim_1)
  pipeline53/1(q) -> [cwg0_tp0], bus_mult/1(a)
  pipeline165/1(q) -> wng1/2(rst)
  Logical21/1 -> pipeline165/1(d)
  man_rst_wng1/1(in_rst) -> [wng_man_rst1], Logical21/2
  [wng_rst0] -> Logical21/1
  Constant100/1 -> man_rst_wng1/1(sim_1)
  pipeline166/1(q) -> wng_corr/2(rst)
  Logical24/1 -> pipeline166/1(d)
  man_rst_wng_corr/1(in_rst) -> [wng_man_rst_corr], Logical24/2
  [wng_rst0] -> Logical24/1
  Constant101/1 -> man_rst_wng_corr/1(sim_1)
  Gateway Out3/1 -> To Workspace3/1
  Gateway Out5/1 -> To Workspace5/1
  bus_convert1/1(dout) -> [cwg1_tp2], pipeline157/1(d)
  Gateway Out6/1 -> To Workspace6/1
  Gateway Out17/1 -> To Workspace17/1
  Constant106/1 -> cwg0/6(en)
  pipeline95/1(q) -> [cwg0], bus_expand2/1(bus_in)
  cwg0/2(dvalid) -> Terminator30/1
  [wng_sum0] -> Delay139/1
  [cwg_corr_out0] -> Delay5/1
  [cwg0] -> bus_addsub2/1(a)
  [cwg_corr_out1] -> Delay86/1
  Constant37/1 -> scale_cwg0/1(sim_1)
  Constant36/1 -> freq_cwg1/1(sim_1)
  scale_cwg1/1(in_scale) -> pipeline44/1(d)
  freq_cwg1/1(in_frequency) -> pipeline52/1(d)
  pipeline52/1(q) -> cwg1/1(freq)
  pipeline44/1(q) -> cwg1/2(scale)
  [mrst] -> pipeline41/1(d)
  Constant33/1 -> rpt_length_cwg1/1(sim_1)
  rpt_en_cwg1/1(in_en) -> Convert1/1
  Constant41/1 -> rpt_en_cwg1/1(sim_1)
  Convert1/1 -> pipeline42/1(d)
  cwg1/1(bus_out) -> pipeline89/1(d)
  rpt_length_cwg1/1(in_repeat_length) -> pipeline43/1(d)
  pipeline41/1(q) -> cwg1/3(rst)
  pipeline42/1(q) -> cwg1/4(repeat_en)
  pipeline43/1(q) -> cwg1/5(repeat_length)
  cwg1/3(rpt_rst) -> Terminator29/1
  Constant23/1 -> cwg1/6(en)
  pipeline89/1(q) -> [cwg1]
  cwg1/2(dvalid) -> Terminator28/1
  Constant30/1 -> scale_cwg1/1(sim_1)
  Constant35/1 -> scale_wng0/1(sim_1)
  pipeline90/1(q) -> [cwg_corr]
  [cwg1] -> bus_addsub3/1(a)
  bus_addsub3/1(dout) -> Delay2/1
  Delay2/1 -> bus_convert5/1(din)
  [cwg_corr] -> bus_addsub3/2(b)
  [wng_sum1] -> Delay9/1
  bus_addsub1/1(dout) -> Delay6/1
  Delay6/1 -> bus_convert3/1(din)
  bus_addsub/1(dout) -> Delay7/1
  Delay7/1 -> bus_convert2/1(din)
  Mux6/1 -> [data_80_1]
  [wng_scale0] -> wng0/1(scale_16_14)
  pipeline198/1(q) -> wng0/2(rst)
  wng0/1(bus_out) -> [wng0_tp0]
  [wng_scale1] -> wng1/1(scale_16_14)
  [wng_scale_corr] -> wng_corr/1(scale_16_14)
  wng1/1(bus_out) -> [wng1_tp0]
  wng_corr/1(bus_out) -> [wng_corr_tp0]
  Gateway Out19/1 -> To Workspace11/1
  Gateway Out20/1 -> To Workspace12/1
  Gateway Out21/1 -> To Workspace14/1
  Gateway Out22/1 -> To Workspace15/1
  Gateway Out23/1 -> To Workspace16/1
  Gateway Out27/1 -> To Workspace18/1
  Constant61/1 -> control/2(sim_2)
  Constant44/1 -> control/3(sim_3)
  Constant60/1 -> control/1(sim_1)
  Constant63/1 -> control/4(sim_4)
  Constant71/1 -> control/5(sim_5)
  Constant72/1 -> control/6(sim_6)
  Constant74/1 -> control/7(sim_7)
  Constant75/1 -> control/8(sim_8)
  Constant76/1 -> control/9(sim_9)
  Gateway Out31/1 -> To Workspace30/1
  Gateway Out28/1 -> To Workspace21/1
  Gateway Out29/1 -> To Workspace29/1
  Gateway Out30/1 -> To Workspace28/1
  bus_expand3/1(msb_out8) -> Gateway Out28/1
  bus_expand3/2(out7) -> Gateway Out31/1
  bus_expand3/4(out5) -> Gateway Out30/1
  bus_expand3/3(out6) -> Gateway Out29/1
  bus_expand3/8(lsb_out1) -> Gateway Out34/1
  bus_expand3/7(out2) -> Gateway Out33/1
  bus_expand3/6(out3) -> Gateway Out35/1
  bus_expand3/5(out4) -> Gateway Out32/1
  Gateway Out34/1 -> To Workspace20/1
  Gateway Out33/1 -> To Workspace22/1
  Gateway Out35/1 -> To Workspace23/1
  Gateway Out32/1 -> To Workspace27/1
  [cwg_80_0] -> bus_expand3/1(bus_in)
  Gateway Out39/1 -> To Workspace37/1
  Gateway Out36/1 -> To Workspace31/1
  Gateway Out37/1 -> To Workspace36/1
  Gateway Out38/1 -> To Workspace35/1
  bus_expand4/1(msb_out8) -> Gateway Out36/1
  bus_expand4/2(out7) -> Gateway Out39/1
  bus_expand4/4(out5) -> Gateway Out38/1
  bus_expand4/3(out6) -> Gateway Out37/1
  bus_expand4/8(lsb_out1) -> Gateway Out42/1
  bus_expand4/7(out2) -> Gateway Out41/1
  bus_expand4/6(out3) -> Gateway Out43/1
  bus_expand4/5(out4) -> Gateway Out40/1
  Gateway Out42/1 -> To Workspace19/1
  Gateway Out41/1 -> To Workspace32/1
  Gateway Out43/1 -> To Workspace33/1
  Gateway Out40/1 -> To Workspace34/1
  [cwg_80_1] -> bus_expand4/1(bus_in)
  Gateway Out47/1 -> To Workspace46/1
  Gateway Out44/1 -> To Workspace39/1
  Gateway Out45/1 -> To Workspace45/1
  Gateway Out46/1 -> To Workspace44/1
  bus_expand5/1(msb_out8) -> Gateway Out44/1
  bus_expand5/2(out7) -> Gateway Out47/1
  bus_expand5/4(out5) -> Gateway Out46/1
  bus_expand5/3(out6) -> Gateway Out45/1
  bus_expand5/8(lsb_out1) -> Gateway Out50/1
  bus_expand5/7(out2) -> Gateway Out49/1
  bus_expand5/6(out3) -> Gateway Out51/1
  bus_expand5/5(out4) -> Gateway Out48/1
  Gateway Out50/1 -> To Workspace40/1
  Gateway Out49/1 -> To Workspace41/1
  Gateway Out51/1 -> To Workspace42/1
  Gateway Out48/1 -> To Workspace43/1
  bus_expand6/1(msb_out8) -> Gateway Out52/1
  bus_expand6/2(out7) -> Gateway Out55/1
  bus_expand6/4(out5) -> Gateway Out54/1
  bus_expand6/3(out6) -> Gateway Out53/1
  bus_expand6/8(lsb_out1) -> Gateway Out58/1
  bus_expand6/7(out2) -> Gateway Out57/1
  bus_expand6/6(out3) -> Gateway Out59/1
  bus_expand6/5(out4) -> Gateway Out56/1
  Gateway Out58/1 -> To Workspace47/1
  Gateway Out57/1 -> To Workspace48/1
  Gateway Out59/1 -> To Workspace49/1
  Gateway Out56/1 -> To Workspace50/1
  Gateway Out54/1 -> To Workspace51/1
  Gateway Out55/1 -> To Workspace53/1
  Gateway Out53/1 -> To Workspace52/1
  Gateway Out52/1 -> To Workspace54/1
  Gateway Out60/1 -> To Workspace2/1
  Gateway Out61/1 -> To Workspace55/1
  Gateway Out62/1 -> To Workspace56/1
  Gateway Out63/1 -> To Workspace57/1
  Gateway Out64/1 -> To Workspace58/1
  Gateway Out65/1 -> To Workspace59/1
  Gateway Out66/1 -> To Workspace60/1
  Gateway Out67/1 -> To Workspace61/1
  Gateway Out68/1 -> To Workspace62/1
  Gateway Out69/1 -> To Workspace63/1
  Gateway Out70/1 -> To Workspace64/1
  Gateway Out71/1 -> To Workspace65/1
  Gateway Out72/1 -> To Workspace66/1
  Gateway Out73/1 -> To Workspace67/1
  Gateway Out74/1 -> To Workspace68/1
  Gateway Out75/1 -> To Workspace69/1
  Gateway Out76/1 -> To Workspace70/1
  Gateway Out77/1 -> To Workspace71/1
  Gateway Out78/1 -> To Workspace72/1
  pipeline107/1(q) -> Logical49/2, Gateway Out78/1, pack_80_64_2/4(pkt_start)
  Gateway Out79/1 -> To Workspace73/1
  Gateway Out80/1 -> To Workspace74/1
  Gateway Out81/1 -> To Workspace75/1
  Gateway Out82/1 -> To Workspace76/1
  Gateway Out83/1 -> To Workspace77/1
  Gateway Out84/1 -> To Workspace78/1
  Gateway Out85/1 -> To Workspace79/1
  Gateway Out86/1 -> To Workspace80/1
  Gateway Out87/1 -> To Workspace81/1
  Gateway Out88/1 -> To Workspace82/1
  Gateway Out89/1 -> To Workspace83/1
  Gateway Out90/1 -> To Workspace84/1
  Gateway Out91/1 -> To Workspace85/1
  Gateway Out92/1 -> To Workspace86/1
  Gateway Out93/1 -> To Workspace87/1
  Gateway Out94/1 -> To Workspace88/1
  Gateway Out95/1 -> To Workspace89/1
  Gateway Out96/1 -> To Workspace90/1
  Gateway Out97/1 -> To Workspace91/1
  Gateway Out98/1 -> To Workspace92/1
  Gateway Out99/1 -> To Workspace93/1
  Gateway Out100/1 -> To Workspace94/1
  Constant10/1 -> Terminator/1
  Constant12/1 -> Terminator32/1
  Constant13/1 -> Terminator33/1
  Constant14/1 -> Terminator34/1
  64_to_3/2 -> Mux17/3, bram_munge3/1(In1)
  64_to_1/2 -> Mux16/3, bram_munge2/1(In1)
  64_to_2/2 -> Mux18/3, bram_munge1/1(In1)
  pipeline74/1(q) -> pipeline75/1(d), edge_detect17/1(in)
  64_to_256/2 -> Mux19/3, bram_munge0/1(In1)
  master_reset_sim10/1 -> ramp_control/1(sim_1)
  master_reset_sim11/1 -> ramp_control/2(sim_2)
  master_reset_sim12/1 -> ramp_control/3(sim_3)
  master_reset_sim13/1 -> ramp_control/4(sim_4)
  Gateway Out107/1 -> To Workspace102/1
  Gateway Out108/1 -> To Workspace111/1
  Gateway Out109/1 -> To Workspace112/1
  Gateway Out110/1 -> To Workspace113/1
  Mux21/1 -> Gateway Out110/1, spead_pack3/3(data64)
  Gateway Out113/1 -> To Workspace114/1
  [sp256_dv] -> pipeline226/1(d), edge_detect33/1, pipeline208/1(d)
  [gbe_txip] -> pipeline194/1(d)
  [sp256_eof] -> pipeline196/1(d)
  pipeline194/1(q) -> ss_ip_tx/1(in_ip)
  pipeline196/1(q) -> ss_ip_tx/2(in_eof)
  pipeline208/1(q) -> ss_ip_tx/3(in_dv)
  pipeline226/1(q) -> ss_ip_tx/4(we)
  pipeline230/1(q) -> ss_ip_tx/5(trig)
  edge_detect33/1 -> pipeline230/1(d)
  [sp256_dv0] -> Mux2/1
  [sp256_data0] -> Mux2/3
  [sp256_data2] -> Mux2/2
  [sp256_dv1] -> pipeline14/1(d)
  Mux2/1 -> Mux7/2
  [sp256_data1] -> pipeline186/1(d)
  [sp256_dv3] -> pipeline16/1(d)
  Mux7/1 -> Mux8/2
  [sp256_data3] -> pipeline187/1(d)
  Mux8/1 -> pipeline193/1(d)
  pipeline186/1(q) -> Mux7/3
  pipeline187/1(q) -> pipeline188/1(d)
  pipeline188/1(q) -> Mux8/3
  [sp256_dvg0] -> Logical38/1
  [sp256_dvg1] -> Logical38/2
  [sp256_dvg2] -> Logical38/3
  [sp256_dvg3] -> Logical38/4
  Logical38/1 -> pipeline229/1(d)
  pipeline229/1(q) -> pipeline231/1(d)
  pipeline231/1(q) -> pipeline169/1(d)
  [sp256_eofg0] -> Logical10/1
  [sp256_eofg2] -> Logical10/3
  Logical10/1 -> pipeline232/1(d)
  pipeline232/1(q) -> pipeline9/1(d)
  pipeline9/1(q) -> pipeline175/1(d)  "tx_eof"
  pipeline14/1(q) -> Mux7/1
  pipeline16/1(q) -> pipeline66/1(d)
  pipeline66/1(q) -> Mux8/1
  Gateway Out4/1 -> To Workspace9/1
  Gateway Out9/1 -> To Workspace4/1
  Gateway Out12/1 -> To Workspace7/1
  Gateway Out15/1 -> To Workspace8/1
  bus_expand1/1(msb_out4) -> Gateway Out15/1
  bus_expand1/2(out3) -> Gateway Out4/1
  Gateway Out16/1 -> To Workspace10/1
  bus_expand1/3(out2) -> Gateway Out16/1
  Gateway Out18/1 -> To Workspace38/1
  bus_expand1/4(lsb_out1) -> Gateway Out18/1
  Concat11/1 -> pipeline164/1(d)
  pipeline164/1(q) -> pipeline168/1(d)
  [sp256_dv1] -> edge_detect15/1(in), Concat11/2
  Constant104/1 -> Mux4/2
  [gbe_ip1] -> Mux4/3
  Concat12/1 -> pipeline69/1(d)
  pipeline69/1(q) -> pipeline153/1(d)
  [gbe_ip0] -> Mux24/3
  Constant103/1 -> Mux24/2
  [sp256_dv2] -> edge_detect16/1(in), Concat12/1
  [sp256_dv0] -> edge_detect28/1(in), Concat12/2
  [gbe_ip2] -> Mux24/4
  Constant105/1 -> Mux24/5
  [gbe_ip3] -> Mux4/4
  Constant102/1 -> Mux4/5
  pipeline153/1(q) -> pipeline174/1(d), Mux31/1, Mux30/1, Mux12/1, Mux24/1
  Gateway Out105/1 -> To Workspace99/1
  Concat13/1 -> Gateway Out106/1, Mux27/1
  Slice5/1 -> Logical51/1
  Slice6/1 -> Logical51/2
  Slice7/1 -> Logical52/1
  Slice8/1 -> Logical52/2
  Constant114/1 -> Mux27/2
  Constant128/1 -> Mux27/5
  Logical51/1 -> Concat13/2, Logical64/1
  Logical52/1 -> Concat13/1, Logical64/2
  Mux4/1 -> Mux13/2
  pipeline173/1(q) -> Slice5/1, Slice6/1
  pipeline174/1(q) -> Slice8/1, Slice7/1
  Gateway Out106/1 -> To Workspace100/1
  [gbe_ip0] -> Relational15/2
  [gbe_ip1] -> Relational16/2
  [gbe_ip2] -> Relational17/2
  [gbe_ip3] -> Relational18/2
  ip_count0/1(sim_out) -> To Workspace101/1
  Counter9/1 -> ip_count0/1(out_ip_count0)
  Counter12/1 -> ip_count3/1(out_ip_count3)
  Gateway Out111/1 -> To Workspace105/1
  Gateway Out112/1 -> To Workspace106/1
  Gateway Out114/1 -> To Workspace108/1
  Gateway Out115/1 -> To Workspace109/1
  Gateway Out116/1 -> To Workspace110/1
  Counter11/1 -> ip_count2/1(out_ip_count2)
  Counter10/1 -> ip_count1/1(out_ip_count1)
  ip_count1/1(sim_out) -> To Workspace103/1
  ip_count2/1(sim_out) -> To Workspace104/1
  ip_count3/1(sim_out) -> To Workspace107/1
  Relational15/1 -> Logical53/1
  Relational16/1 -> Logical54/1
  Logical53/1 -> Gateway Out112/1, Counter9/2
  Logical54/1 -> Counter10/2, Gateway Out114/1
  Logical55/1 -> Counter11/2, Gateway Out115/1
  Relational18/1 -> Logical56/1
  Logical56/1 -> Counter12/2, Gateway Out116/1
  pipeline168/1(q) -> Mux29/1, Mux28/1, Mux11/1, Mux4/1, pipeline173/1(d)
  [sp256_eofg1] -> Logical10/2
  [sp256_eofg3] -> Logical10/4
  [sp256_eofg0] -> pipeline183/1(d)
  pipeline183/1(q) -> Logical53/2
  [sp256_eofg1] -> pipeline184/1(d)
  [sp256_eofg2] -> pipeline185/1(d)
  [sp256_eofg3] -> pipeline192/1(d)
  pipeline184/1(q) -> Logical54/2
  pipeline185/1(q) -> Logical55/2
  pipeline192/1(q) -> Logical56/2
  Relational17/1 -> Logical55/1
  [sp256_dv3] -> edge_detect14/1(in), Concat11/1
  edge_detect14/1(out) -> Logical57/1
  edge_detect15/1(out) -> Logical57/2
  Logical57/1 -> Delay91/1
  Register/1 -> Gateway Out122/1, Mux27/3
  Register4/1 -> Gateway Out101/1, Mux27/4
  edge_detect16/1(out) -> Logical58/1
  edge_detect28/1(out) -> Logical58/2
  Logical58/1 -> Delay88/1
  Delay88/1 -> Delay89/1
  Delay89/1 -> Delay87/1
  Delay90/1 -> Delay97/1
  Delay91/1 -> Delay92/1
  Delay92/1 -> Delay90/1
  Mux27/1 -> Gateway Out129/1, Register7/1
  Register7/1 -> Gateway Out105/1, [gbe_txip]
  edge_detect30/1(out) -> Logical59/1
  edge_detect31/1(out) -> Logical59/2
  Logical59/1 -> Register7/2, Gateway Out130/1
  Gateway Out129/1 -> To Workspace127/1
  Gateway Out130/1 -> To Workspace128/1
  edge_detect32/1(out) -> Logical59/4
  edge_detect29/1(out) -> Logical59/3
  [sp256_dv0] -> Delay96/1
  [sp256_dv2] -> Delay95/1
  [sp256_dv1] -> Delay94/1
  [sp256_dv3] -> Delay93/1
  Delay93/1 -> edge_detect30/1(in)
  Delay94/1 -> edge_detect31/1(in)
  Delay95/1 -> edge_detect29/1(in)
  Delay96/1 -> edge_detect32/1(in)
  pipeline169/1(q) -> Gateway Out9/1, [sp256_dv]
  pipeline175/1(q) -> Gateway Out12/1, [sp256_eof]
  pipeline193/1(q) -> bus_expand1/1(bus_in), [sp256_data]
  Counter16/1 -> ip_count4/1(out_ip_count0)
  Counter15/1 -> ip_count7/1(out_ip_count3)
  Counter14/1 -> ip_count6/1(out_ip_count2)
  Counter13/1 -> ip_count5/1(out_ip_count1)
  ip_count4/1(sim_out) -> To Workspace115/1
  ip_count5/1(sim_out) -> To Workspace116/1
  ip_count6/1(sim_out) -> To Workspace117/1
  ip_count7/1(sim_out) -> To Workspace1/1
  Logical63/1 -> Counter15/2
  Logical62/1 -> Counter14/2
  Logical61/1 -> Counter13/2
  Logical60/1 -> Counter16/2
  Relational19/1 -> Logical60/1
  Relational20/1 -> Logical61/1
  Relational21/1 -> Logical62/1
  Relational22/1 -> Logical63/1
  pipeline262/1(q) -> Logical60/2
  pipeline263/1(q) -> Logical61/2
  pipeline265/1(q) -> Logical62/2
  pipeline266/1(q) -> Logical63/2
  [gbe_ip4] -> Relational19/2
  [gbe_ip5] -> Relational20/2
  [gbe_ip6] -> Relational21/2
  [gbe_ip7] -> Relational22/2
  Constant136/1 -> Mux11/2
  Constant137/1 -> Mux11/5
  [gbe_ip5] -> Mux11/3
  [gbe_ip7] -> Mux11/4
  Constant138/1 -> Mux12/2
  Constant139/1 -> Mux12/5
  [gbe_ip4] -> Mux12/3
  [gbe_ip6] -> Mux12/4
  Mux13/1 -> Register/1, Gateway Out120/1
  Mux11/1 -> Mux13/3
  [ip_range_sel] -> Mux13/1
  Logical64/1 -> edge_detect36/1(in)
  edge_detect36/1(out) -> Counter17/2
  [msync] -> Counter17/1
  Counter17/1 -> Slice14/1, Gateway Out104/1
  Gateway Out104/1 -> To Workspace118/1
  Gateway Out117/1 -> To Workspace119/1
  [sp256_eofg3] -> pipeline266/1(d)
  [sp256_eofg2] -> pipeline265/1(d)
  [sp256_eofg1] -> pipeline263/1(d)
  [sp256_eofg0] -> pipeline262/1(d)
  Gateway Out118/1 -> To Workspace120/1
  Gateway Out119/1 -> To Workspace121/1
  Gateway Out120/1 -> To Workspace122/1
  Gateway Out121/1 -> To Workspace125/1
  Gateway Out122/1 -> To Workspace126/1
  Delay97/1 -> Gateway Out121/1, Register/2
  Mux12/1 -> Mux26/3
  Mux26/1 -> Gateway Out102/1, Register4/1
  Delay98/1 -> Register4/2
  Delay87/1 -> Delay98/1
  Gateway Out101/1 -> To Workspace95/1
  Gateway Out102/1 -> To Workspace96/1
  Constant149/1 -> Mux28/2
  Constant150/1 -> Mux28/5
  [gbe_ip9] -> Mux28/3
  [gbe_ip11] -> Mux28/4
  Constant151/1 -> Mux29/2
  Constant152/1 -> Mux29/5
  [gbe_ip13] -> Mux29/3
  [gbe_ip15] -> Mux29/4
  Mux28/1 -> Gateway Out118/1, Mux13/4
  Mux29/1 -> Gateway Out119/1, Mux13/5
  Slice14/1 -> Gateway Out117/1, [ip_range_sel]
  pipeline10/1(q) -> [gbe_ip3]
  pipeline11/1(q) -> [gbe_ip2]
  pipeline13/1(q) -> [gbe_ip0]
  pipeline12/1(q) -> [gbe_ip1]
  gbe_iptx0/1(in_reg) -> pipeline13/1(d)
  gbe_iptx1/1(in_reg) -> pipeline12/1(d)
  gbe_iptx2/1(in_reg) -> pipeline11/1(d)
  gbe_iptx3/1(in_reg) -> pipeline10/1(d)
  Constant98/1 -> gbe_iptx3/1(sim_1)
  Constant84/1 -> gbe_iptx2/1(sim_1)
  Constant83/1 -> gbe_iptx1/1(sim_1)
  Constant78/1 -> gbe_iptx0/1(sim_1)
  pipeline207/1(q) -> [gbe_ip7]
  pipeline227/1(q) -> [gbe_ip6]
  pipeline261/1(q) -> [gbe_ip4]
  pipeline228/1(q) -> [gbe_ip5]
  gbe_iptx4/1(in_reg) -> pipeline261/1(d)
  gbe_iptx5/1(in_reg) -> pipeline228/1(d)
  gbe_iptx6/1(in_reg) -> pipeline227/1(d)
  gbe_iptx7/1(in_reg) -> pipeline207/1(d)
  Constant135/1 -> gbe_iptx7/1(sim_1)
  Constant134/1 -> gbe_iptx6/1(sim_1)
  Constant130/1 -> gbe_iptx5/1(sim_1)
  Constant129/1 -> gbe_iptx4/1(sim_1)
  pipeline267/1(q) -> [gbe_ip11]
  pipeline268/1(q) -> [gbe_ip10]
  pipeline270/1(q) -> [gbe_ip8]
  pipeline269/1(q) -> [gbe_ip9]
  gbe_iptx8/1(in_reg) -> pipeline270/1(d)
  gbe_iptx9/1(in_reg) -> pipeline269/1(d)
  gbe_iptx10/1(in_reg) -> pipeline268/1(d)
  gbe_iptx11/1(in_reg) -> pipeline267/1(d)
  Constant148/1 -> gbe_iptx11/1(sim_1)
  Constant147/1 -> gbe_iptx10/1(sim_1)
  Constant146/1 -> gbe_iptx9/1(sim_1)
  Constant145/1 -> gbe_iptx8/1(sim_1)
  pipeline271/1(q) -> [gbe_ip15]
  pipeline275/1(q) -> [gbe_ip14]
  pipeline277/1(q) -> [gbe_ip12]
  pipeline276/1(q) -> [gbe_ip13]
  gbe_iptx12/1(in_reg) -> pipeline277/1(d)
  gbe_iptx13/1(in_reg) -> pipeline276/1(d)
  gbe_iptx14/1(in_reg) -> pipeline275/1(d)
  gbe_iptx15/1(in_reg) -> pipeline271/1(d)
  Constant144/1 -> gbe_iptx15/1(sim_1)
  Constant143/1 -> gbe_iptx14/1(sim_1)
  Constant142/1 -> gbe_iptx13/1(sim_1)
  Constant141/1 -> gbe_iptx12/1(sim_1)
  Mux24/1 -> Mux26/2
  Constant85/1 -> Mux30/2
  Constant140/1 -> Mux30/5
  [gbe_ip8] -> Mux30/3
  [gbe_ip10] -> Mux30/4
  Constant154/1 -> Mux31/2
  Constant153/1 -> Mux31/5
  [gbe_ip12] -> Mux31/3
  [gbe_ip14] -> Mux31/4
  Mux30/1 -> Mux26/4
  Mux31/1 -> Mux26/5
  [ip_range_sel] -> Mux26/1
  Counter20/1 -> ip_count8/1(out_ip_count0)
  Counter19/1 -> ip_count11/1(out_ip_count3)
  Counter18/1 -> ip_count10/1(out_ip_count2)
  Counter2/1 -> ip_count9/1(out_ip_count1)
  Logical31/1 -> Counter19/2
  Logical30/1 -> Counter18/2
  Logical29/1 -> Counter2/2
  Logical28/1 -> Counter20/2
  Relational12/1 -> Logical28/1
  Relational23/1 -> Logical29/1
  Relational24/1 -> Logical30/1
  Relational25/1 -> Logical31/1
  pipeline240/1(q) -> Logical28/2
  pipeline241/1(q) -> Logical29/2
  pipeline242/1(q) -> Logical30/2
  pipeline243/1(q) -> Logical31/2
  [gbe_ip8] -> Relational12/2
  [gbe_ip9] -> Relational23/2
  [gbe_ip10] -> Relational24/2
  [gbe_ip11] -> Relational25/2
  [sp256_eofg3] -> pipeline243/1(d)
  [sp256_eofg2] -> pipeline242/1(d)
  [sp256_eofg1] -> pipeline241/1(d)
  [sp256_eofg0] -> pipeline240/1(d)
  ip_count8/1(sim_out) -> To Workspace124/1
  ip_count9/1(sim_out) -> To Workspace97/1
  ip_count10/1(sim_out) -> To Workspace98/1
  ip_count11/1(sim_out) -> To Workspace129/1
  Counter24/1 -> ip_count14/1(out_ip_count0)
  Counter22/1 -> ip_count13/1(out_ip_count3)
  Counter21/1 -> ip_count12/1(out_ip_count2)
  Counter23/1 -> ip_count15/1(out_ip_count1)
  Logical35/1 -> Counter22/2
  Logical34/1 -> Counter21/2
  Logical33/1 -> Counter23/2
  Logical32/1 -> Counter24/2
  [msync] -> Counter20/1, Counter2/1, Counter18/1, Counter22/1, Counter21/1, Counter23/1, Counter24/1, Counter19/1, Counter15/1, Counter14/1, Counter13/1, Counter16/1, Counter12/1, Counter11/1, Counter10/1, Counter9/1, Gateway Out111/1
  Relational26/1 -> Logical32/1
  Relational27/1 -> Logical33/1
  Relational28/1 -> Logical34/1
  Relational29/1 -> Logical35/1
  [gbe_txip] -> Relational20/1, Relational12/1, Relational24/1, Relational27/1, Relational29/1, Relational28/1, Relational26/1, Relational25/1, Relational23/1, Relational22/1, Relational21/1, Relational19/1, Relational18/1, Relational17/1, Relational16/1, Relational15/1
  pipeline244/1(q) -> Logical32/2
  pipeline245/1(q) -> Logical33/2
  pipeline246/1(q) -> Logical34/2
  pipeline247/1(q) -> Logical35/2
  [gbe_ip12] -> Relational26/2
  [gbe_ip13] -> Relational27/2
  [gbe_ip14] -> Relational28/2
  [gbe_ip15] -> Relational29/2
  [sp256_eofg3] -> pipeline247/1(d)
  [sp256_eofg2] -> pipeline246/1(d)
  [sp256_eofg1] -> pipeline245/1(d)
  [sp256_eofg0] -> pipeline244/1(d)
  ip_count14/1(sim_out) -> To Workspace130/1
  ip_count15/1(sim_out) -> To Workspace131/1
  ip_count13/1(sim_out) -> To Workspace133/1
  ip_count12/1(sim_out) -> To Workspace132/1
